simulink model "Simu_Simulink"  (R2016a)
settings: Solver=FixedStepDiscrete  StartTime=0.0  StopTime=20  FixedStep=0.01  RelTol=1e-3
InitFcn:
  |     if ~coder.target('MATLAB')
  | coder.ceval('NMPC_Solve_initialize');
  |     end
values from neighbouring files (symbols this model uses):
  p = zeros(OCP.dim.p,solverOptions.N)    [CodeGen.m]    (also in Simu_Matlab.m)
  Ts = 0.01    [Simu_Matlab.m]
  x0 = [0,0,0,0,0,0,0,0,0].'    [CodeGen.m]    (also in Simu_Matlab.m = sysSimu(uOpt,x0,p(:,1),Ts,10))
settings Model: Creator=Deng  LastModifiedBy=deng
settings OptimizationCC: ZeroExternalMemoryAtStartup=off  SimCompilerOptimization=on
settings HardwareCC: ProdWordSize=32  ProdHWDeviceType=Specified
settings SFSimCC: SimUserSources=NMPC_Solve.cpp init_solution.cpp timer_unix.cpp NMPC_Solve_WithInitSolution.cpp  SimUserIncludeDirs=./quadrotor_codegen ./quadrotor_codegen/simulink  SimParseCustomCode=off
settings RTWCC: GenerateReport=on  RTWUseSimCustomCode=on  CustomInclude=./quadrotor_codegen ./quadrotor_codegen/simulink  CustomSource=NMPC_Solve.cpp init_solution.cpp timer_unix.cpp NMPC_Solve_WithInitSolution.cpp  BuildConfiguration=Faster Runs  LaunchReport=on  TargetLang=C++
settings GRTTargetCC: TargetLangStandard=C++03 (ISO)  MultiInstanceERTCode=on  CodeInterfacePackaging=C++ class

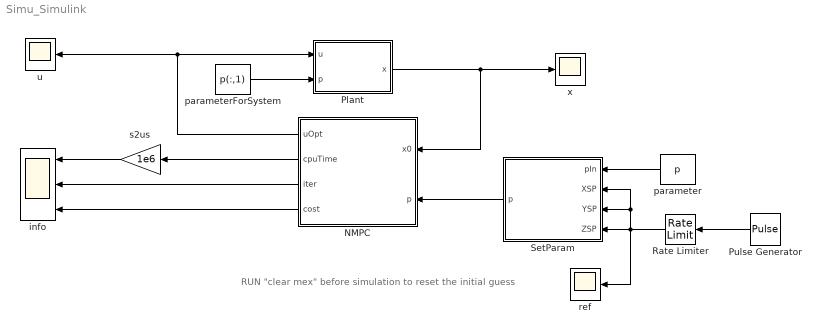
== system Simu_Simulink ==
  note: RUN "clear mex" before simulation to reset the initial guess
  NMPC : Subsystem
  Plant : Subsystem
  Pulse Generator : DiscretePulseGenerator  PulseType=Time based  Amplitude=2  Period=20  PulseWidth=50  PhaseDelay=5
  Rate Limiter : RateLimiter  RisingSlewLimit=5  FallingSlewLimit=-5  SampleTimeMode=inherited
  SetParam : MATLAB Function  TreatAsAtomicUnit=on
  info : Scope  NumInputPorts=3
  parameter : Constant  Value=p  VectorParams1D=off
  parameterForSystem : Constant  Value=p(:,1)  VectorParams1D=off
  ref : Scope
  s2us : Gain  Gain=1e6
  u : Scope
  x : Scope
  wires:
  Plant/1(x) -> x/1, NMPC/1(x0)
  NMPC/1(uOpt) -> Plant/1(u), u/1
  NMPC/2(cpuTime) -> s2us/1
  s2us/1 -> info/1
  NMPC/3(iter) -> info/2
  NMPC/4(cost) -> info/3
  Pulse Generator/1 -> Rate Limiter/1
  parameter/1 -> SetParam/1(pIn)
  Rate Limiter/1 -> SetParam/3(YSP), SetParam/2(XSP), ref/1, SetParam/4(ZSP)
  SetParam/1(p) -> NMPC/2(p)
  parameterForSystem/1 -> Plant/2(p)

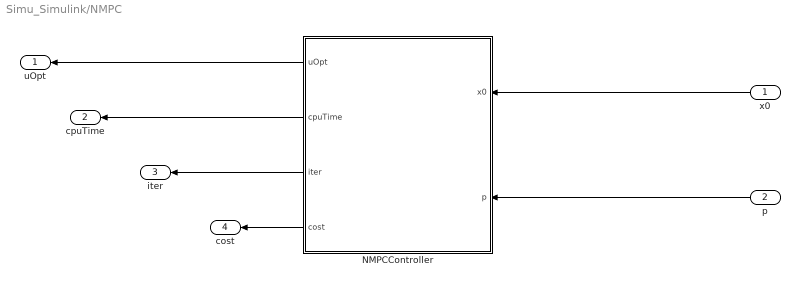
== system Simu_Simulink/NMPC ==
  x0 : Inport
  p : Inport  Port=2
  NMPCController : MATLAB Function  TreatAsAtomicUnit=on
  uOpt : Outport
  cpuTime : Outport  Port=2
  iter : Outport  Port=3
  cost : Outport  Port=4
  wires:
  p/1 -> NMPCController/2(p)
  x0/1 -> NMPCController/1(x0)
  NMPCController/1(uOpt) -> uOpt/1
  NMPCController/2(cpuTime) -> cpuTime/1
  NMPCController/4(cost) -> cost/1
  NMPCController/3(iter) -> iter/1

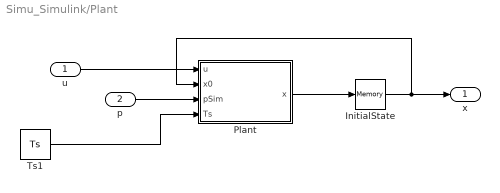
== system Simu_Simulink/Plant ==
  u : Inport
  p : Inport  Port=2
  InitialState : Memory  X0=x0
  Plant : MATLAB Function  TreatAsAtomicUnit=on
  Ts1 : Constant  Value=Ts
  x : Outport
  wires:
  Plant/1(x) -> InitialState/1
  InitialState/1 -> Plant/2(x0), x/1
  u/1 -> Plant/1(u)
  Ts1/1 -> Plant/4(Ts)
  p/1 -> Plant/3(pSim)

== matlab function Simu_Simulink/Plant/Plant ==
  data: u input; x0 input; pSim input; x output; Ts input
function x = plant(u,x0,pSim,Ts)%#codegen

x = sysSimu(u,x0,pSim,Ts,10);

== matlab function Simu_Simulink/SetParam ==
  data: pIn input; XSP input; YSP input; ZSP input; p output
function p = SetParam(pIn,XSP,YSP,ZSP)
%#codegen
p = pIn;
p(1,:) = XSP;
p(2,:) = YSP;
p(3,:) = ZSP;

== matlab function Simu_Simulink/NMPC/NMPCController ==
  data: x0 input; p input; uOpt output; cpuTime output; iter output; cost output
function [uOpt,cpuTime,iter,cost]  = NMPC(x0,p)%#codegen
solverOptions = createSolverOptions();
coder.cstructname(solverOptions, 'SolverOptions', 'extern', 'HeaderFile', 'NMPC_Solve_types.h');

solverOptions.T      = 1;
solverOptions.N      = 20;

[solution_c,output]  = NMPC_Solve_Wrapper_Simulink(x0,p,solverOptions);
coder.cstructname(solution_c, 'Solution', 'extern', 'HeaderFile', 'NMPC_Solve_types.h');
coder.cstructname(output,'Output', 'extern', 'HeaderFile', 'NMPC_Solve_types.h'); 
%%
uOpt    = solution_c.u(:,1);
cpuTime = output.cpuTime;
iter = output.iterations;
cost = output.cost;
end

%%
% output      = createOutput();
% solution    = createNonemptySolution();
% 
% % call the generated function
% coder.ceval('NMPC_Solve',...
%              x0,...
%              p,...
%              coder.wref(solution),...
%              coder.wref(output));
% 
% uOptimal = solution.u(1:4,1);
% cpuTime  = output.timeElapsed.total;
% KKTError = output.KKTError;
% iter     = output.iterTotal;
% cost     = output.cost;
